simulink model "Kalman_filter_conv"  (R2019a)
settings: Solver=FixedStepDiscrete  StartTime=0.0  StopTime=10.0  FixedStep=0.2  RelTol=1e-3  EnableMultiTasking=on
undefined symbols (not defined in the file): DiscIntNeverNeededParam
settings Model: Creator=PC  LastModifiedBy=administrator
settings OptimizationCC: EnhancedBackFolding=on  PassReuseOutputArgsAs=Individual arguments  MaxStackSize=64  OptimizeBlockOrder=speed  DifferentSizesBufferReuse=on  OptimizationCustomize=off
settings DebuggingCC: ParameterTunabilityLossMsg=error
settings HardwareCC: ProdBitPerPointer=32  ProdBitPerSizeT=32  ProdBitPerPtrDiffT=32  ProdLargestAtomicInteger=Long  ProdLargestAtomicFloat=Double  ProdWordSize=32  ProdHWDeviceType=ARM Compatible->ARM Cortex
settings SFSimCC: MATLABDynamicMemAlloc=off
settings RTWCC: SystemTargetFile=ert.tlc  GenCodeOnly=on  TemplateMakefile=ert_default_tmf  GenerateReport=on  Toolchain=GNU Tools for ARM Embedded Processors  IncludeHyperlinkInReport=on  LaunchReport=on  TargetLang=C++  GenerateTraceInfo=on  GenerateTraceReport=on  GenerateTraceReportSl=on  GenerateTraceReportSf=on  GenerateTraceReportEml=on
settings CodeAppCC: ForceParamTrailComments=on  IgnoreCustomStorageClasses=off  OperatorAnnotations=on  SimulinkDataObjDesc=on  SFDataObjDesc=on  InsertBlockDesc=on
settings ERTTargetCC: TargetLangStandard=C++03 (ISO)  MultiInstanceERTCode=on  CodeInterfacePackaging=Reusable function  RootIOFormat=Structure reference  ERTCustomFileTemplate=example_file_process.tlc

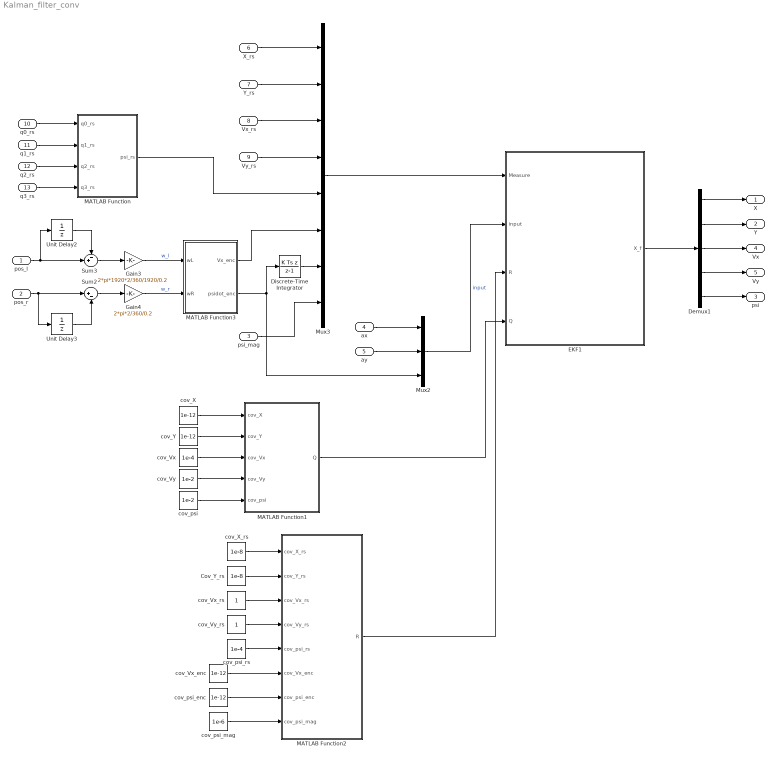
== system Kalman_filter_conv ==
  pos_l : Inport
  pos_r : Inport  Port=2
  psi_mag : Inport  Port=3
  ax : Inport  Port=4
  ay : Inport  Port=5
  X_rs : Inport  Port=6
  Y_rs : Inport  Port=7
  Vx_rs : Inport  Port=8
  Vy_rs : Inport  Port=9
  q0_rs : Inport  Port=10
  q1_rs : Inport  Port=11
  q2_rs : Inport  Port=12
  q3_rs : Inport  Port=13
  Cov_Y_rs : Constant  Value=1e-8
  Demux1 : Demux  Outputs=5
  Discrete-Time Integrator : DiscreteIntegrator  IntegratorMethod=Integration: Backward Euler  SampleTime=-1  ICPrevOutput=DiscIntNeverNeededParam  ICPrevScaledInput=DiscIntNeverNeededParam
  EKF1 : Subsystem
  Gain3 : Gain  Gain=2*pi*1920*2/360/1920/0.2
  Gain4 : Gain  Gain=2*pi*2/360/0.2
  MATLAB Function : MATLAB Function  TreatAsAtomicUnit=on
  MATLAB Function1 : MATLAB Function  TreatAsAtomicUnit=on
  MATLAB Function2 : MATLAB Function  TreatAsAtomicUnit=on
  MATLAB Function3 : MATLAB Function  TreatAsAtomicUnit=on
  Mux2 : Mux  Inputs=3
  Mux3 : Mux  Inputs=8
  Sum2 : Sum  Inputs=|+-
  Sum3 : Sum  Inputs=-+|
  Unit Delay2 : UnitDelay  SampleTime=-1  HasFrameUpgradeWarning=on
  Unit Delay3 : UnitDelay  SampleTime=-1  HasFrameUpgradeWarning=on
  cov_Vx : Constant  Value=1e-4
  cov_Vx_enc : Constant  Value=1e-12
  cov_Vx_rs : Constant
  cov_Vy : Constant  Value=1e-2
  cov_Vy_rs : Constant
  cov_X : Constant  Value=1e-12
  cov_X_rs : Constant  Value=1e-8
  cov_Y : Constant  Value=1e-12
  cov_psi : Constant  Value=1e-2
  cov_psi_enc : Constant  Value=1e-12
  cov_psi_mag : Constant  Value=1e-6
  cov_psi_rs : Constant  Value=1e-4
  X : Outport  VectorParamsAs1DForOutWhenUnconnected=on
  Y : Outport  Port=2  VectorParamsAs1DForOutWhenUnconnected=on
  "psi " : Outport  Port=3  VectorParamsAs1DForOutWhenUnconnected=on
  "Vx " : Outport  Port=4  VectorParamsAs1DForOutWhenUnconnected=on
  "Vy " : Outport  Port=5  VectorParamsAs1DForOutWhenUnconnected=on
  wires:
  psi_mag/1 -> Mux3/8
  cov_Vx/1 -> MATLAB Function1/3(cov_Vx)
  MATLAB Function1/1(Q) -> EKF1/4(Q)
  cov_X/1 -> MATLAB Function1/1(cov_X)
  cov_Vy/1 -> MATLAB Function1/4(cov_Vy)
  cov_psi/1 -> MATLAB Function1/5(cov_psi)
  cov_Y/1 -> MATLAB Function1/2(cov_Y)
  q1_rs/1 -> MATLAB Function/2(q1_rs)
  q3_rs/1 -> MATLAB Function/4(q3_rs)
  q2_rs/1 -> MATLAB Function/3(q2_rs)
  MATLAB Function/1(psi_rs) -> Mux3/5
  Demux1/5 -> "psi "/1
  Demux1/4 -> "Vy "/1
  X_rs/1 -> Mux3/1
  MATLAB Function3/1(Vx_enc) -> Mux3/6
  Y_rs/1 -> Mux3/2
  Vx_rs/1 -> Mux3/3
  Demux1/3 -> "Vx "/1
  ay/1 -> Mux2/2
  Discrete-Time Integrator/1 -> Mux3/7
  Unit Delay2/1 -> Sum3/1
  ax/1 -> Mux2/1
  Demux1/1 -> X/1
  Mux3/1 -> EKF1/1(Measure)
  pos_l/1 -> Unit Delay2/1, Sum3/2
  Gain3/1 -> MATLAB Function3/1(wL)  "w_l"
  MATLAB Function3/2(psidot_enc) -> Discrete-Time Integrator/1, Mux2/3
  Mux2/1 -> EKF1/2(input)  "input"
  Sum3/1 -> Gain3/1
  EKF1/1(X_f) -> Demux1/1
  Demux1/2 -> Y/1
  Gain4/1 -> MATLAB Function3/2(wR)  "w_r"
  Sum2/1 -> Gain4/1
  q0_rs/1 -> MATLAB Function/1(q0_rs)
  MATLAB Function2/1(R) -> EKF1/3(R)
  pos_r/1 -> Sum2/1, Unit Delay3/1
  Unit Delay3/1 -> Sum2/2
  Vy_rs/1 -> Mux3/4
  cov_Vx_rs/1 -> MATLAB Function2/3(cov_Vx_rs)
  cov_psi_enc/1 -> MATLAB Function2/7(cov_psi_enc)
  cov_Vy_rs/1 -> MATLAB Function2/4(cov_Vy_rs)
  Cov_Y_rs/1 -> MATLAB Function2/2(cov_Y_rs)
  cov_psi_rs/1 -> MATLAB Function2/5(cov_psi_rs)
  cov_psi_mag/1 -> MATLAB Function2/8(cov_psi_mag)
  cov_X_rs/1 -> MATLAB Function2/1(cov_X_rs)
  cov_Vx_enc/1 -> MATLAB Function2/6(cov_Vx_enc)

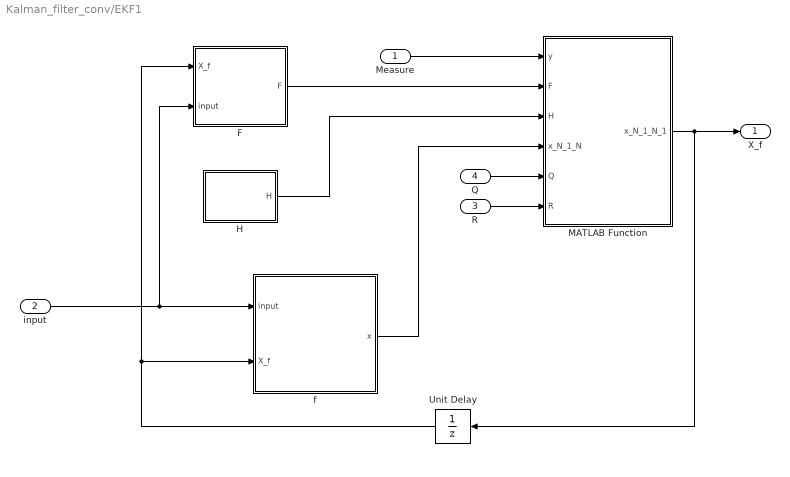
== system Kalman_filter_conv/EKF1 ==
  Measure : Inport
  input : Inport  Port=2
  R : Inport  Port=3
  Q : Inport  Port=4
  F : MATLAB Function  TreatAsAtomicUnit=on
  H : MATLAB Function  TreatAsAtomicUnit=on
  MATLAB Function : MATLAB Function  TreatAsAtomicUnit=on
  Unit Delay : UnitDelay  InitialCondition=[0 0 0 0 0]  SampleTime=-1  HasFrameUpgradeWarning=on
  f : MATLAB Function  TreatAsAtomicUnit=on
  X_f : Outport  VectorParamsAs1DForOutWhenUnconnected=on
  wires:
  Measure/1 -> MATLAB Function/1(y)
  MATLAB Function/1(x_N_1_N_1) -> Unit Delay/1, X_f/1
  F/1(F) -> MATLAB Function/2(F)
  H/1(H) -> MATLAB Function/3(H)
  Q/1 -> MATLAB Function/5(Q)
  R/1 -> MATLAB Function/6(R)
  f/1(x) -> MATLAB Function/4(x_N_1_N)
  Unit Delay/1 -> f/2(X_f), F/1(X_f)
  input/1 -> F/2(input), f/1(input)

== matlab function Kalman_filter_conv/MATLAB Function1 ==
  data: cov_X input; Q output; cov_Y input; cov_Vx input; cov_Vy input; cov_psi input
function Q = fcn(cov_X, cov_Y, cov_Vx, cov_Vy, cov_psi)

Q=[cov_X    0     0       0         0;...
    0     cov_Y   0       0         0;...
    0       0    cov_Vx   0         0;...
    0       0     0     cov_Vy      0;...
    0       0     0       0      cov_psi];

== matlab function Kalman_filter_conv/MATLAB Function ==
  data: q0_rs input; psi_rs output; q1_rs input; q2_rs input; q3_rs input
function psi_rs = fcn(q0_rs, q1_rs, q2_rs, q3_rs)

psi_rs= atan2(2*(q0_rs*q3_rs+q1_rs*q2_rs),1-2*(q2_rs^2+q3_rs^2));

== matlab function Kalman_filter_conv/MATLAB Function2 ==
  data: cov_X_rs input; R output; cov_Y_rs input; cov_Vx_rs input; cov_Vy_rs input; cov_psi_rs input; cov_Vx_enc input; cov_psi_enc input; cov_psi_mag input
function R = fcn(cov_X_rs, cov_Y_rs, cov_Vx_rs, cov_Vy_rs, cov_psi_rs, cov_Vx_enc, cov_psi_enc, cov_psi_mag)






R=eye(8,8);

R(1,1)=cov_X_rs;
R(2,2)=cov_Y_rs;
R(3,3)=cov_Vx_rs;
R(4,4)=cov_Vy_rs;
R(5,5)=cov_psi_rs;
R(6,6)=cov_Vx_enc;
R(7,7)=cov_psi_enc;
R(8,8)=cov_psi_mag;

== matlab function Kalman_filter_conv/EKF1/F ==
  data: X_f input; F output; input input
function F = fcn(X_f,input)

F=zeros(5,5);
X=X_f(1);
Y=X_f(2);
Vx=X_f(3);
Vy=X_f(4);
psi=X_f(5);

omega=input(3);

dt=0.2;

F=[1 0 dt*cos(psi) dt*(-sin(psi)) (-Vx*sin(psi)-cos(psi)*Vy)*dt; ...
   0 1 dt*sin(psi) dt*cos(psi) (cos(psi)*Vx-sin(psi)*Vy)*dt; ...
   0 0 1 omega*dt 0; ...
   0 0 -omega*dt 1 0; ...
   0 0 0 0 1];

== matlab function Kalman_filter_conv/EKF1/H ==
  data: H output
function H = fcn()

H=[1 0 0 0 0 ;...
   0 1 0 0 0 ;...
   0 0 1 0 0 ;...
   0 0 0 1 0 ;...
   0 0 0 0 1 ;...
   0 0 1 0 0 ;...
   0 0 0 0 1 ;...
   0 0 0 0 1 ];

== matlab function Kalman_filter_conv/EKF1/MATLAB Function ==
  data: y input; x_N_1_N_1 output; F input; H input; x_N_1_N input; Q input; R input
function x_N_1_N_1  = fcn(y, F, H, x_N_1_N, Q, R)

x_N_1_N_1=zeros(5,1);

persistent P_N_N

if isempty(P_N_N)
    P_N_N = eye(5);
end

% A priori estimation
x_N_1_N;

% A priori estimate error covariance matrix
P_N_1_N = F*P_N_N*F' + Q; 

% Filter gain
K = P_N_1_N*H'/(H*P_N_1_N*H' + R); 

% Innovation
err = y - H*x_N_1_N;  

% Update of state estimation
x_N_1_N_1 = x_N_1_N + K*err; 

% Update of covariance error matrix
P_N_1_N_1 = (eye(5) - K*H)*P_N_1_N; 

P_N_N = P_N_1_N_1;

== matlab function Kalman_filter_conv/EKF1/f ==
  data: input input; x output; X_f input
function x = fcn(input, X_f)
dt=0.2;

X=X_f(1);
Y=X_f(2);
Vx=X_f(3);
Vy=X_f(4);
psi=X_f(5);

ax=input(1);
ay=input(2);
omega=input(3);

dX= X+(cos(psi)*Vx-sin(psi)*Vy)*dt;
dY= Y+(sin(psi)*Vx+cos(psi)*Vy)*dt;
dVx=Vx+(ax+omega*Vy)*dt;
dVy=Vy+(ay-omega*Vx)*dt;
dpsi=omega*dt+psi;


x=[dX, dY, dVx, dVy, dpsi]';

== matlab function Kalman_filter_conv/MATLAB Function3 ==
  data: wL input; Vx_enc output; wR input; psidot_enc output
function [Vx_enc,psidot_enc] = fcn(wL,wR)
r=0.043/2;
B=0.185;

Vx_enc=r/2*(wR+wL);
psidot_enc=r/B*(wR-wL);
